simulink model "rudder_sensors"  (Simulink 7.5)
settings: Solver=FixedStepDiscrete  SolverMode=SingleTasking  StartTime=0.0  StopTime=10.0  FixedStep=0.01  RelTol=1e-3
libraries: dsPICdrivers x7, simulink x1
settings Model: Creator=Bryant  LastModifiedBy=Bryant
settings OptimizationCC: OptimizeModelRefInitCode=on  LifeSpan=1
settings HardwareCC: ProdBitPerInt=16  ProdEndianess=LittleEndian  ProdWordSize=16  ProdHWDeviceType=16-bit Generic
settings RTWCC: SystemTargetFile=dspic.tlc  MakeCommand=make_CreateMPLAB  TemplateMakefile=dspic_pic30_gcc.tmf  PostCodeGenCommand=dsPIC_Compile()  Description=Embedded Target for Microchip dsPIC (real-time)  ProcessScript=dspic_make_rtw_hook
settings CodeAppCC: IgnoreCustomStorageClasses=off
settings STFCustomTargetCC: IncludeMdlTerminateFcn=off  CombineOutputUpdateFcns=on  SuppressErrorStatus=on  ERTCustomFileBanners=on  SupportContinuousTime=off  SupportNonInlinedSFcns=off  SystemTargetFile=dspic.tlc
settings ERTTargetCC: MultiwordLength=2048  ParMdlRefBuildCompliant=off  CompOptLevelCompliant=off  IncludeMdlTerminateFcn=off  SuppressErrorStatus=on  ERTFirstTimeCompliant=off  ModelStepFunctionPrototypeControlCompliant=off  CPPClassGenCompliant=off  ExtModeMexFile=ext_serial_win32_comm  InlinedParameterPlacement=NonHierarchical  ERTSrcFileBannerTemplate=dsPIC_code_template.cgt  ERTHdrFileBannerTemplate=dsPIC_code_template.cgt  ERTDataSrcFileTemplate=dsPIC_code_template.cgt  ERTDataHdrFileTemplate=dsPIC_code_template.cgt  ERTCustomFileTemplate=dsPIC_main.tlc  ConvertIfToSwitch=off
settings CustomProperty: DataType=string  Value=C:\PROGRA~1\MATLAB\R2010a\bin\win64\gmake

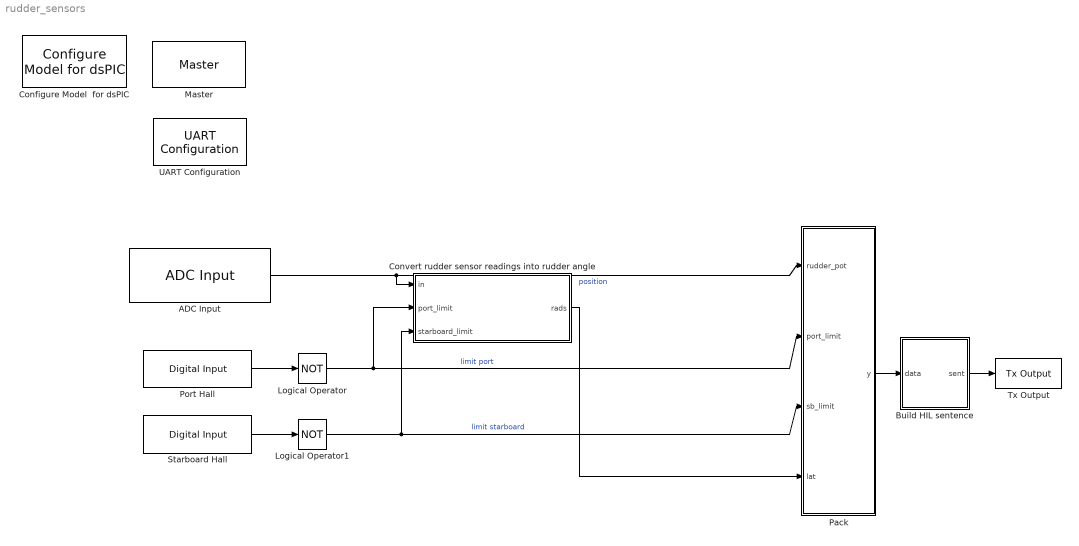
== system rudder_sensors ==
  ADC Input : dsPICdrivers/Peripheral I//O/ADC Input  Tag=dsPIC_ADC  Priority=5  ADC_TYPE=10 bits  ADC_MODE=Continuous sampling & get last channel value  NbrSampleStep=1  VoltRefpopup="AVdd  -  AVss"  OutFormatBitspopup=0000 00dd dddd dddd : Integer  InterruptPriority=6  ANCHANNELS=[0]  MaxName=ANmax = 1023  Rin=1e2  ADCS=12  SAMC=1  Temperature=25  DMAChannel=7  SampleTime=0.01  Status="OK  |  Tsmp=1.625e-007 |  T/Channel=2.113e-006 |  Tall=2.113e-006"  SSRC=auto convert
  Build HIL sentence : Subsystem
  Configure Model  for dsPIC : dsPICdrivers/Simulink Configuration/Configure Model  for dsPIC
  Convert rudder sensor readings into rudder angle : Stateflow chart  TreatAsAtomicUnit=on
  Logical Operator : Logic  Operator=NOT  Inputs=1  AllPortsSameDT=off  OutDataTypeMode=boolean  LogicDataType=fixdt(0, 8)  OutDataTypeStr=boolean
  Logical Operator1 : Logic  Operator=NOT  Inputs=1  AllPortsSameDT=off  OutDataTypeMode=boolean  LogicDataType=fixdt(0, 8)  OutDataTypeStr=boolean
  Master : dsPICdrivers/Master  Tag=dsPIC_MASTER  Priority=1  TimeStepType=Timer1  picType=33fJ256GP710  fcy=40000000  Quartz_33f=8e6  PLLActive_33f=on  fcyDesired_33f=40000000  tmr1="[8  49999  0]"  tmr1Info="Time Step : 0.01  ;   Error : 0%  PR1=49999"  tmr2345="[0  0  0  0  0  0  0  0]"  tmr2345cfg=[-1 -1 -1 -1 -1 -1 -1 -1]  IOautoConf=on  typePort="[ 0  0  0  0  0  0  0  0  0  0  0  0  0  0  0  0  8  0  0  0  0  0  0  0  0  0  0  0  0  0  0  0  0  0  9  0  0  0  0  0  0  0  0  0  0  0  0  0  0  0  0  0  0  0  0  0  0  0  0  0  0  0  0  0  0  0  0  0  0  0  0  0  0  0  0  0  0  0  0  0  0  0  4  5  0  0  0  0  0  0  0  0  0  0  0  0  0  0  0  9  0  0  0  0  0  0  0  0  0  0  0  0 ]"  TRIS="[ 65535  65535  65535  65535  65535  65535  65535 ]"  ADPCFG=131072  MasterBusyPort=None  MasterOverloadPort=None  FOSC=Quartz (XT - HS)  ClockSwitchMonitor=Both disabled  TempProtection_33f=TEMP_ON  FPBOR=<empty>  PWRT=disable  MCLR=<empty>  ICD=ICS_PGD1  JTAGEN=JTAGEN_OFF  PowerSave=off  OverrideFcy=off  NewFcy=1e6  PR2345="[65535  65535  65535  65535  65535  65535  65535  65535]"
  Pack : Stateflow chart  TreatAsAtomicUnit=on
  Port Hall : dsPICdrivers/Digital I//O/Digital Input  Tag=dsPIC_Digital_Input  PORT=C  Pin=[2]  SampleTime=.01  OrderingInOutPopup=None
  Starboard Hall : dsPICdrivers/Digital I//O/Digital Input  Tag=dsPIC_Digital_Input  PORT=G  Pin=[3]  SampleTime=.01  OrderingInOutPopup=None
  Tx Output : dsPICdrivers/Serial PORT/Tx Output  Tag=dsPIC_TX  Priority=5  UART=1  OrderingInOutPopup=None
  UART Configuration : dsPICdrivers/Serial PORT/UART Configuration  Tag=dsPIC_config_UART  Priority=2  UART=1  proposed_BAUD=115200  BAUD=115200  ALT_TX_RX=off  InterruptTxWhen=When Transmit Buffer is empty  TXInterruptPri=1  TxBufferSize=32  TXEN=on  InterruptRxWhen=When Receive Buffer is full (contain 4 characters)  RXInterruptPri=2  RxBufferSize=32  DoNotImplementRxInterrupt=off  DoNotImplementTxInterrupt=off  UxBRG=21  Info="UxBRG = 21   ||  Real Baud : 113636   ||  % error : -1.3573  ||  max 113.6364 Bytes / Step"  RealBaud=0  ERROR=-1.3573  BYTES_STEP=113.6364
  wires:
  ADC Input/1 -> Convert rudder sensor readings into rudder angle/1(in), Pack/1(rudder_pot)  "position"
  Port Hall/1 -> Logical Operator/1
  Logical Operator/1 -> Convert rudder sensor readings into rudder angle/2(port_limit), Pack/2(port_limit)  "limit port"
  Convert rudder sensor readings into rudder angle/1(rads) -> Pack/4(lat)
  Starboard Hall/1 -> Logical Operator1/1
  Logical Operator1/1 -> Convert rudder sensor readings into rudder angle/3(starboard_limit), Pack/3(sb_limit)  "limit starboard"
  Pack/1(y) -> Build HIL sentence/1(data)
  Build HIL sentence/1(sent) -> Tx Output/1

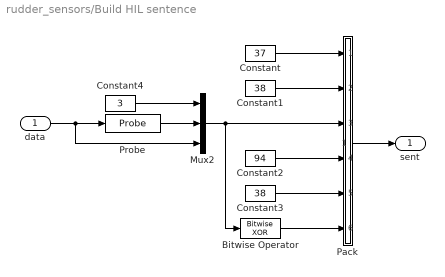
== system rudder_sensors/Build HIL sentence ==
  data : Inport
  Bitwise Operator : simulink/Logic and Bit Operations/Bitwise Operator  logicop=XOR  UseBitMask=off  BitMask=bin2dec('11011001')  BitMaskRealWorld=Stored Integer
  Constant : Constant  Value=37  OutDataTypeMode=uint8  OutDataType=fixdt(1, 16)  OutScaling=2^0  OutDataTypeStr=uint8
  Constant1 : Constant  Value=38  OutDataTypeMode=uint8  OutDataType=fixdt(1, 16)  OutScaling=2^0  OutDataTypeStr=uint8
  Constant2 : Constant  Value=94  OutDataTypeMode=uint8  OutDataType=fixdt(1, 16)  OutScaling=2^0  OutDataTypeStr=uint8
  Constant3 : Constant  Value=38  OutDataTypeMode=uint8  OutDataType=fixdt(1, 16)  OutScaling=2^0  OutDataTypeStr=uint8
  Constant4 : Constant  Value=3  OutDataTypeMode=uint8  OutDataType=fixdt(1, 16)  OutScaling=2^0  OutDataTypeStr=uint8
  Mux2 : Mux  Inputs=3
  Pack : Stateflow chart  TreatAsAtomicUnit=on
  Probe : Probe  ProbeSampleTime=off  ProbeComplexSignal=off  ProbeWidthDataType=uint8
  sent : Outport
  wires:
  data/1 -> Probe/1, Mux2/3
  Constant/1 -> Pack/1(a)
  Constant1/1 -> Pack/2(b)
  Pack/1(y) -> sent/1
  Mux2/1 -> Bitwise Operator/1, Pack/3(c)
  Probe/1 -> Mux2/2
  Constant2/1 -> Pack/4(d)
  Constant3/1 -> Pack/5(e)
  Bitwise Operator/1 -> Pack/6(f)
  Constant4/1 -> Mux2/1

== matlab function Convert rudder sensor readings into rudder angle ==
  data: in input uint16; rads output single; port_limit input boolean; starboard_limit input boolean
function rads = pot_to_rads(in, port_limit, starboard_limit)
%#eml

persistent low_side high_side lastInput offset
if isempty(low_side) || isempty(high_side)
    low_side = int32(-1);
    high_side = int32(-1);
    lastInput = int32(-10000);
    offset = int32(0);
end

% Here we track transitions. On a high->low transition start adding 1023
% and on a low->high transition don't add anything. It "centers" the input
% range around 1023.
input = int32(in);
if lastInput == uint32(-10000)
    lastInput = input;
end
jump = input - lastInput;
if jump > 1000
    offset = int32(0);
elseif jump < -1000
    offset = int32(1023);
end

% We record the last input BEFORE it's offset. This fixes situations where
% we're comparing data before and after the very first transition.
lastInput = input;

% Apply any offset that should be there.
input = input + offset;

% Update port range limit when the Hall limit switch. Only update to the
% maximum value obtained during the limit switch active period.
if port_limit && (input > high_side || high_side == -1)
    high_side = input;
    
    % If the high_side limit is less than the low_side one, we add 1023
    % assuming that it's a valid value (ie. ~= -1).
    if high_side < low_side && high_side ~= -1
        high_side = high_side + 1023;
    end
end

% Update starboard ADC value when limit is reached. Only update to the
% maximum value obtained during the limit switch active period.
if starboard_limit && (input < low_side || low_side == -1)
    low_side = input;
    
    % If the high_side limit is less than the low_side one, we add 1023
    % assuming that it's a valid value (ie. ~= -1).
    if high_side < low_side && high_side ~= -1
        high_side = high_side + 1023;
    end
end

% Return 0 when we can't actually determine the rudder position
if high_side == -1 || low_side == -1
    rads = single(0);
    return;
end

% Prepare our input. Here we subtract the baseline 'low_side' value off of
% the input so we start with a range from [0..high_side-lowside] and map it
% into the output range of 45 degrees.
in_min = 0;
in_max = high_side - low_side;
out_min = int32(-45);
out_max = int32(45);
val = input - low_side;

% This is a basic integer implementation of a map() function. It was pulled
% from: http://www.arduino.cc/cgi-bin/yabb2/YaBB.pl?num=1289758376, first
% post.
% NOTE: There can be integer overflow in the first multiplication, but with
% the set of inputs we're seeing here the maximum value of the multiplication
% is 90*1023 = 92070, far below intmax32.
mappedValue = (val - in_min) * (out_max - out_min) / (in_max - in_min) + out_min;

% Finally convert to radians and a double before returning it.
rads = single(mappedValue) * pi / 180;

== matlab function Pack ==
  data: y output double; rudder_pot input double; port_limit input double; sb_limit input double; lat input double
function y = fcn(rudder_pot, port_limit, sb_limit, lat)
%#eml

y = zeros(97, 1, 'uint8');
y(53:54) = packUint16BE(rudder_pot);
y(55) = port_limit;
y(56) = sb_limit;
y(57:60) = packUint32BE(typecast(lat,'uint32'));

function out = packUint32BE(in)
out = zeros(4, 1, 'uint8');
out(1) = uint8(bitand(bitshift(in,-24),hex2dec('FF')));
out(2) = uint8(bitand(bitshift(in,-16),hex2dec('FF')));
out(3) = uint8(bitand(bitshift(in,-8),hex2dec('FF')));
out(4) = uint8(bitand(in,hex2dec('FF')));

function out = packUint16BE(in)
out = zeros(2, 1, 'uint8');
out(1) = uint8(bitand(bitshift(in,-8),hex2dec('FF')));
out(2) = uint8(bitand(in,hex2dec('FF')));

== matlab function Build HIL sentence/Pack ==
  data: a input double; y output double; b input double; c input double; d input double; e input double; f input double
function y = fcn(a, b, c, d, e, f)
%#eml

y = zeros(length(a)+length(b)+length(c)+length(d)+length(e)+length(f), 1, 'uint8');
y(1) = a;
y(2) = b;
y(3:101) = c;
y(102) = d;
y(103) = e;
y(104) = f;
